simulink model "state_feedback_no_estimator"  (R2015b)
settings: Solver=VariableStepAuto  StartTime=0.0  StopTime=20.0  RelTol=1e-3
values from neighbouring files (symbols this model uses):
  A = [zeros(2) eye(2); -inv(M)*kappa -inv(M)*beta]    [Lab3_Solution.m]    (also in lab4.m = [0 0 1 0; 0 0 0 1; 0 (mp^2 * l^2 *g)/mu (-c*Jt)/mu (-Y*Jt*l*; lab4_pid_controller.m; lab4_state_feedback_no_estimator.m; lab4_state_feedback_with_estimator.m)
  B = [0; 0; inv(M)*S]    [Lab3_Solution.m]    (also in lab4.m = [0; 0; Jt/mu; (l*mp)/mu]; lab4_pid_controller.m; lab4_state_feedback_no_estimator.m; lab4_state_feedback_with_estimator.m)
  C = [1 0 0 0; 0 1 0 0]    [Lab3_Solution.m]    (also in PendulumTutorial.m = zpk(z,p,k); lab4.m; lab4_pid_controller.m = eye(4); lab4_state_feedback_no_estimator.m = eye(4))
  D = [0; 0]    [Lab3_Solution.m]    (also in lab4.m; lab4_pid_controller.m = [0; 0; 0; 0]; lab4_state_feedback_no_estimator.m = [0; 0; 0; 0]; lab4_state_feedback_with_estimator.m)
  K = 20    [PendulumTutorial.m]    (also in lab4_state_feedback_no_estimator.m = place(A,B,p); lab4_state_feedback_with_estimator.m = place(A,B,p))
  kr = -1/(C*inv(A-B*K)*B)    [lab4_state_feedback_no_estimator.m]    (also in lab4_state_feedback_with_estimator.m)
settings Model: Creator=lukasgemar  LastModifiedBy=Lukas Gemar

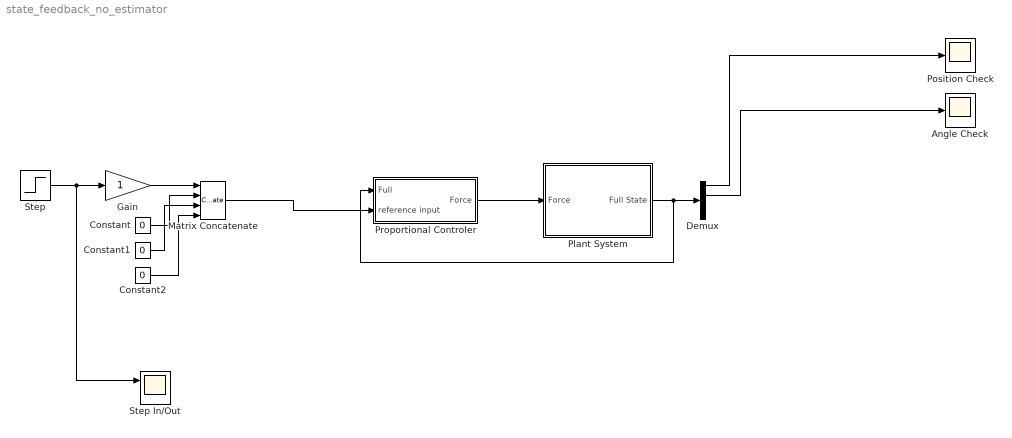
== system state_feedback_no_estimator ==
  Angle Check : Scope
  Constant : Constant  Value=0
  Constant1 : Constant  Value=0
  Constant2 : Constant  Value=0
  Demux : Demux
  Gain : Gain
  Matrix Concatenate : Concatenate  NumInputs=4  Mode=Multidimensional array
  Plant System : Subsystem
  Position Check : Scope
  Proportional Controler : Subsystem
  Step : Step  SampleTime=0
  "Step In/Out " : Scope  NumInputPorts=2
  wires:
  Step/1 -> Gain/1, "Step In/Out "/1
  Proportional Controler/1(Force) -> Plant System/1(Force)
  Plant System/1(Full State) -> Proportional Controler/1(Full), Demux/1
  Gain/1 -> Matrix Concatenate/1
  Constant/1 -> Matrix Concatenate/2
  Constant1/1 -> Matrix Concatenate/3
  Constant2/1 -> Matrix Concatenate/4
  Matrix Concatenate/1 -> Proportional Controler/2(reference input)
  Demux/1 -> Position Check/1
  Demux/2 -> Angle Check/1

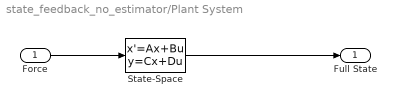
== system state_feedback_no_estimator/Plant System ==
  Force : Inport
  State-Space : StateSpace  A=A  B=B  C=C  D=D  X0=[0;0;0;0]
  Full State : Outport
  wires:
  Force/1 -> State-Space/1
  State-Space/1 -> Full State/1

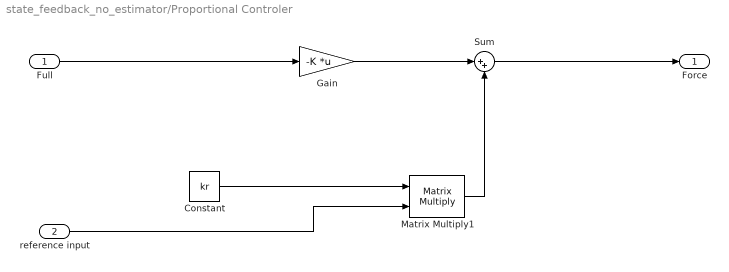
== system state_feedback_no_estimator/Proportional Controler ==
  Full : Inport
  reference input : Inport  Port=2
  Constant : Constant  Value=kr  VectorParams1D=off
  Gain : Gain  Gain=-K  Multiplication=Matrix(K*u)
  Matrix Multiply1 : Product  Multiplication=Matrix(*)
  Sum : Sum  Inputs=|++
  Force : Outport
  wires:
  Gain/1 -> Sum/1
  Sum/1 -> Force/1
  Matrix Multiply1/1 -> Sum/2
  Constant/1 -> Matrix Multiply1/1
  reference input/1 -> Matrix Multiply1/2
  Full/1 -> Gain/1
